simulink model "sampleModel1528"  (R2023a)
settings: Solver=VariableStepAuto  StartTime=0.0  StopTime=10.0  RelTol=1e-3
libraries: hdlsllib x5, simulink x1
settings Model: Creator=user1  LastModifiedBy=user1

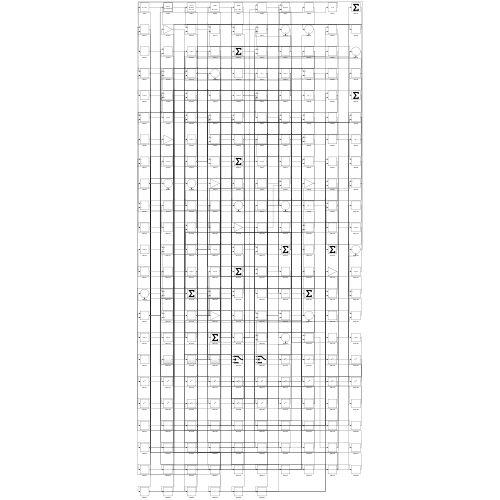
[thumbnail: Simulink's stored preview of the top-level diagram]
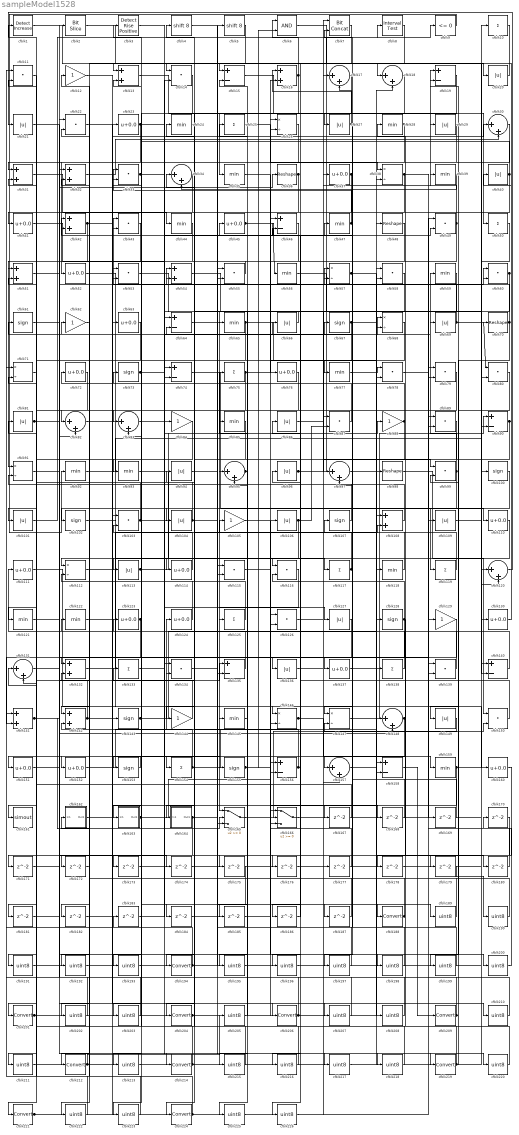
== system sampleModel1528 ==
  cfblk1 : simulink/Logic and Bit Operations/Detect Increase  vinit=0.0  OutDataTypeStr=boolean
      settings: LibrarySourceBlock=|
      | hdlsllib/Logic and Bit
      | Operations/Detect
      | Increase
  cfblk{10,25,50,75,117,119,125,133,138,154} (10 alike) : Sum  Inputs=+
  cfblk{61,67,73,100,102,107,128,143,153,155} (10 alike) : Signum
  cfblk{20..21,27,29,40,66,69,81,86,94,96,101,104,106,109,113,127,136,149} (19 alike) : Abs  SaturateOnIntegerOverflow=off
  cfblk{11,14,22,33,43,49,53,55,58,60,78..80,87,89,99,103,115..116,126,134,139,150} (23 alike) : DotProduct  OutDataTypeStr=Inherit: Inherit via internal rule
  cfblk{12,62,84,88,105,129,144} (7 alike) : Gain
  cfblk{13,16,31..32,42,51,54,108,132,141..142} (11 alike) : Sum
  cfblk{23,37,41,45,52,63,72,76,110..111,114,123..124,130,137,151..152,160} (18 alike) : Bias  Bias=0.0  SaturateOnIntegerOverflow=off
  cfblk{26,38,57,68,71,91,112,146..147} (9 alike) : Product  Inputs=*/  RndMeth=Zero  SaturateOnIntegerOverflow=on
  cfblk{24,28,35,39,44,47,56,59,65,77,85,92..93,118,121..122,145,159} (18 alike) : MinMax
  cfblk{17..18,30,34,82..83,95,97,120,131,148,157} (12 alike) : Sum  Inputs=|++
  cfblk{15,19,46,64,74,90,135,140,156,158} (10 alike) : Sum  Inputs=+-
  cfblk161 : ToWorkspace  VariableName=simout  SaveFormat=Timeseries  SampleTime=-1
  cfblk162 : Subsystem
      settings: LibrarySourceBlock=|
      | hdlsllib/Ports &
      | Subsystems/Subsystem
  cfblk163 : Subsystem
      settings: LibrarySourceBlock=|
      | hdlsllib/Ports &
      | Subsystems/Subsystem
  cfblk164 : Subsystem
      settings: LibrarySourceBlock=|
      | hdlsllib/Ports &
      | Subsystems/Subsystem
  cfblk165 : Switch  SaturateOnIntegerOverflow=off  InputSameDT=off
  cfblk166 : Switch  SaturateOnIntegerOverflow=off  InputSameDT=off
  cfblk{167..187} (21 alike) : Delay  SampleTime=1
  cfblk{188,194,201,204,206,209,212,214,219,221,224} (11 alike) : DataTypeConversion  SaturateOnIntegerOverflow=off  RndMeth=Floor
  cfblk{189..193,195..200,202..203,205,207..208,210..211,213,215..218,220,222..223,225..226} (28 alike) : DataTypeConversion  OutDataTypeStr=uint8  SaturateOnIntegerOverflow=off  RndMeth=Floor
  cfblk2 : hdlsllib/Logic and Bit Operations/Bit Slice  lidx=7  ridx=0
  cfblk3 : hdlsllib/Logic and Bit Operations/Detect Rise Positive  vinit=0  OutDataTypeStr=boolean
  cfblk{36,48,70,98} (4 alike) : Reshape
  cfblk4 : ArithShift  BitShiftNumber=8
  cfblk5 : ArithShift  BitShiftNumber=8
  cfblk6 : Logic  AllPortsSameDT=off  OutDataTypeStr=boolean
  cfblk7 : hdlsllib/Logic and Bit Operations/Bit Concat  numInputs=2
  cfblk8 : hdlsllib/Logic and Bit Operations/Interval Test  IntervalClosedRight=on  uplimit=0.5  IntervalClosedLeft=on  lowlimit=-0.5  OutDataTypeStr=boolean
  cfblk9 : hdlsllib/Logic and Bit Operations/Compare To Zero  relop=<=  OutDataTypeStr=boolean
  wires:
  cfblk88/1 -> cfblk165/1, cfblk17/2
  cfblk134/1 -> cfblk188/1
  cfblk70/1 -> cfblk43/1, cfblk179/1
  cfblk52/1 -> cfblk117/1
  cfblk13/1 -> cfblk50/1
  cfblk100/1 -> cfblk119/1
  cfblk87/1 -> cfblk72/1
  cfblk101/1 -> cfblk8/1
  cfblk89/1 -> cfblk224/1
  cfblk19/1 -> cfblk83/1
  cfblk9/1 -> cfblk92/1
  cfblk93/1 -> cfblk116/1
  cfblk12/1 -> cfblk63/1
  cfblk158/1 -> cfblk209/1
  cfblk147/1 -> cfblk90/1
  cfblk90/1 -> cfblk13/1, cfblk136/1
  cfblk129/1 -> cfblk194/1
  cfblk96/1 -> cfblk9/1, cfblk99/1
  cfblk98/1 -> cfblk150/1
  cfblk2/1 -> cfblk20/1
  cfblk128/1 -> cfblk141/2, cfblk96/1, cfblk178/1
  cfblk117/1 -> cfblk54/1, cfblk105/1
  cfblk148/1 -> cfblk213/1, cfblk215/1
  cfblk16/1 -> cfblk154/1, cfblk6/1
  cfblk157/1 -> cfblk108/1
  cfblk40/1 -> cfblk137/1, cfblk3/1
  cfblk74/1 -> cfblk110/1
  cfblk115/1 -> cfblk68/1
  cfblk144/1 -> cfblk43/2
  cfblk8/1 -> cfblk18/1
  cfblk29/1 -> cfblk52/1
  cfblk37/1 -> cfblk102/1, cfblk172/1
  cfblk18/1 -> cfblk35/1
  cfblk64/1 -> cfblk95/1
  cfblk41/1 -> cfblk74/1
  cfblk83/1 -> cfblk84/1
  cfblk66/1 -> cfblk65/1
  cfblk47/1 -> cfblk41/1, cfblk33/2
  cfblk113/1 -> cfblk75/1, cfblk88/1, cfblk146/1
  cfblk141/1 -> cfblk165/2, cfblk135/1, cfblk82/2
  cfblk69/1 -> cfblk80/1, cfblk45/1
  cfblk135/1 -> cfblk24/1
  cfblk111/1 -> cfblk145/1
  cfblk136/1 -> cfblk17/1
  cfblk61/1 -> cfblk36/1
  cfblk140/1 -> cfblk111/1
  cfblk120/1 -> cfblk21/1
  cfblk6/1 -> cfblk140/1
  cfblk20/1 -> cfblk14/1
  cfblk26/1 -> cfblk142/1
  cfblk68/1 -> cfblk147/1
  cfblk43/1 -> cfblk91/1
  cfblk156/1 -> cfblk64/2, cfblk46/2
  cfblk130/1 -> cfblk40/1
  cfblk155/1 -> cfblk26/2, cfblk6/2, cfblk60/1
  cfblk11/1 -> cfblk201/1
  cfblk71/1 -> cfblk221/1
  cfblk133/1 -> cfblk219/1
  cfblk154/1 -> cfblk124/1, cfblk18/2, cfblk132/2, cfblk187/1
  cfblk146/1 -> cfblk30/1, cfblk159/1
  cfblk77/1 -> cfblk78/1
  cfblk108/1 -> cfblk91/2
  cfblk165/1 -> cfblk150/2
  cfblk72/1 -> cfblk101/1
  cfblk42/1 -> cfblk161/1, cfblk155/1
  cfblk125/1 -> cfblk42/1
  cfblk104/1 -> cfblk83/2, cfblk220/1
  cfblk166/1 -> cfblk130/1
  cfblk27/1 -> cfblk16/1, cfblk167/1
  cfblk119/1 -> cfblk34/1
  cfblk25/1 -> cfblk38/1
  cfblk59/1 -> cfblk114/1
  cfblk153/1 -> cfblk151/1
  cfblk33/1 -> cfblk68/2, cfblk126/2
  cfblk118/1 -> cfblk95/2
  cfblk35/1 -> cfblk76/1
  cfblk32/1 -> cfblk30/2
  cfblk54/1 -> cfblk138/1
  cfblk143/1 -> cfblk78/2, cfblk55/2, cfblk166/2
  cfblk150/1 -> cfblk86/1
  cfblk75/1 -> cfblk77/1, cfblk144/1
  cfblk1/1 -> cfblk15/1
  cfblk50/1 -> cfblk140/2
  cfblk73/1 -> cfblk67/1, cfblk57/2, cfblk13/2
  cfblk65/1 -> cfblk118/1, cfblk211/1
  cfblk107/1 -> cfblk61/1
  cfblk57/1 -> cfblk157/1, cfblk180/1
  cfblk63/1 -> cfblk121/1
  cfblk80/1 -> cfblk149/1
  cfblk95/1 -> cfblk25/1, cfblk185/1
  cfblk99/1 -> cfblk59/1, cfblk112/1
  cfblk164/1(Out1) -> cfblk108/2, cfblk173/1
  cfblk103/1 -> cfblk5/1, cfblk32/2, cfblk73/1, cfblk31/2
  cfblk142/1 -> cfblk81/1, cfblk29/1
  cfblk22/1 -> cfblk206/1
  cfblk28/1 -> cfblk182/1, cfblk197/1
  cfblk152/1 -> cfblk69/1
  cfblk121/1 -> cfblk2/1
  cfblk36/1 -> cfblk74/2, cfblk135/2
  cfblk159/1 -> cfblk100/1, cfblk166/3
  cfblk10/1 -> cfblk212/1
  cfblk92/1 -> cfblk70/1
  cfblk23/1 -> cfblk127/1, cfblk31/1
  cfblk56/1 -> cfblk90/2
  cfblk53/1 -> cfblk97/1
  cfblk45/1 -> cfblk56/1, cfblk47/1
  cfblk138/1 -> cfblk66/1
  cfblk163/1(Out1) -> cfblk106/1, cfblk57/1, cfblk49/2
  cfblk124/1 -> cfblk12/1
  cfblk116/1 -> cfblk125/1
  cfblk14/1 -> cfblk93/1
  cfblk30/1 -> cfblk163/1(In1)
  cfblk67/1 -> cfblk98/1, cfblk184/1
  cfblk82/1 -> cfblk165/3
  cfblk86/1 -> cfblk37/1
  cfblk49/1 -> cfblk19/1, cfblk104/1, cfblk97/2
  cfblk109/1 -> cfblk120/1
  cfblk114/1 -> cfblk53/2
  cfblk38/1 -> cfblk109/1, cfblk113/1, cfblk226/1
  cfblk31/1 -> cfblk44/1
  cfblk85/1 -> cfblk204/1
  cfblk149/1 -> cfblk147/2
  cfblk44/1 -> cfblk82/1
  cfblk76/1 -> cfblk153/1
  cfblk39/1 -> cfblk34/2
  cfblk97/1 -> cfblk58/1
  cfblk139/1 -> cfblk94/1
  cfblk131/1 -> cfblk214/1
  cfblk15/1 -> cfblk27/1
  cfblk112/1 -> cfblk23/1
  cfblk132/1 -> cfblk46/1
  cfblk81/1 -> cfblk148/2, cfblk60/2
  cfblk123/1 -> cfblk152/1, cfblk33/1
  cfblk24/1 -> cfblk164/1(In1)
  cfblk60/1 -> cfblk54/2, cfblk216/1
  cfblk122/1 -> cfblk87/1
  cfblk21/1 -> cfblk139/2
  cfblk55/1 -> cfblk51/1
  cfblk102/1 -> cfblk160/1
  cfblk126/1 -> cfblk39/1
  cfblk106/1 -> cfblk132/1, cfblk87/2
  cfblk167/1 -> cfblk1/1
  cfblk162/1(Out1) -> cfblk168/1
  cfblk168/1 -> cfblk64/1
  cfblk78/1 -> cfblk169/1
  cfblk169/1 -> cfblk42/2
  cfblk160/1 -> cfblk171/1
  cfblk172/1 -> cfblk142/2
  cfblk173/1 -> cfblk38/2
  cfblk91/1 -> cfblk174/1
  cfblk174/1 -> cfblk26/1
  cfblk145/1 -> cfblk175/1
  cfblk17/1 -> cfblk176/1
  cfblk176/1 -> cfblk148/1
  cfblk177/1 -> cfblk166/1
  cfblk178/1 -> cfblk120/2
  cfblk180/1 -> cfblk139/1
  cfblk84/1 -> cfblk181/1
  cfblk181/1 -> cfblk32/1
  cfblk182/1 -> cfblk14/2
  cfblk183/1 -> cfblk103/2
  cfblk184/1 -> cfblk16/2
  cfblk185/1 -> cfblk156/2
  cfblk48/1 -> cfblk186/1
  cfblk186/1 -> cfblk116/2
  cfblk187/1 -> cfblk15/2
  cfblk188/1 -> cfblk107/1, cfblk162/1(In1)
  cfblk94/1 -> cfblk189/1
  cfblk189/1 -> cfblk134/1
  cfblk179/1 -> cfblk190/1
  cfblk190/1 -> cfblk134/2
  cfblk79/1 -> cfblk191/1
  cfblk191/1 -> cfblk115/1
  cfblk5/1 -> cfblk192/1
  cfblk192/1 -> cfblk79/1
  cfblk46/1 -> cfblk193/1
  cfblk193/1 -> cfblk79/2
  cfblk194/1 -> cfblk115/2, cfblk141/1
  cfblk58/1 -> cfblk195/1
  cfblk195/1 -> cfblk129/1
  cfblk7/1 -> cfblk196/1
  cfblk196/1 -> cfblk80/2
  cfblk197/1 -> cfblk7/1
  cfblk105/1 -> cfblk198/1
  cfblk198/1 -> cfblk7/2
  cfblk170/1 -> cfblk199/1
  cfblk199/1 -> cfblk55/1
  cfblk51/1 -> cfblk200/1
  cfblk200/1 -> cfblk170/1
  cfblk201/1 -> cfblk146/2, cfblk143/1
  cfblk62/1 -> cfblk202/1
  cfblk202/1 -> cfblk11/1
  cfblk175/1 -> cfblk203/1
  cfblk203/1 -> cfblk11/2
  cfblk204/1 -> cfblk58/2, cfblk156/1
  cfblk205/1 -> cfblk85/1
  cfblk206/1 -> cfblk157/2, cfblk126/1
  cfblk171/1 -> cfblk207/1
  cfblk207/1 -> cfblk22/1
  cfblk137/1 -> cfblk208/1
  cfblk208/1 -> cfblk22/2
  cfblk209/1 -> cfblk19/2, cfblk103/1
  cfblk3/1 -> cfblk210/1
  cfblk210/1 -> cfblk158/1
  cfblk211/1 -> cfblk158/2
  cfblk212/1 -> cfblk205/1, cfblk48/1
  cfblk213/1 -> cfblk10/1
  cfblk214/1 -> cfblk112/2, cfblk123/1, cfblk51/2, cfblk122/1
  cfblk215/1 -> cfblk131/1
  cfblk216/1 -> cfblk131/2
  cfblk4/1 -> cfblk217/1
  cfblk217/1 -> cfblk128/1
  cfblk151/1 -> cfblk218/1
  cfblk218/1 -> cfblk4/1
  cfblk219/1 -> cfblk183/1, cfblk99/2, cfblk28/1
  cfblk220/1 -> cfblk133/1
  cfblk221/1 -> cfblk177/1, cfblk53/1
  cfblk34/1 -> cfblk222/1
  cfblk222/1 -> cfblk71/1
  cfblk127/1 -> cfblk223/1
  cfblk223/1 -> cfblk71/2
  cfblk224/1 -> cfblk49/1, cfblk62/1
  cfblk110/1 -> cfblk225/1
  cfblk225/1 -> cfblk89/1
  cfblk226/1 -> cfblk89/2

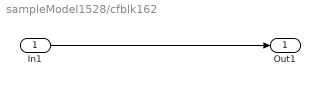
== system sampleModel1528/cfblk162 ==
  In1 : Inport
  Out1 : Outport
  wires:
  In1/1 -> Out1/1

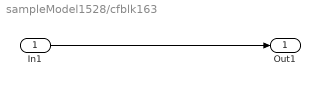
== system sampleModel1528/cfblk163 ==
  In1 : Inport
  Out1 : Outport
  wires:
  In1/1 -> Out1/1

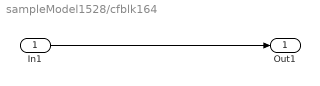
== system sampleModel1528/cfblk164 ==
  In1 : Inport
  Out1 : Outport
  wires:
  In1/1 -> Out1/1
